simulink model "testmodel"  (R2014b)
settings: Solver=ode3  StartTime=0.0  StopTime=10.0  RelTol=1e-3
settings Model: Creator=Bryan  LastModifiedBy=Bryan
settings RTWCC: TemplateMakefile=RTW.MSVCBuild  Description=Create Visual C/C++ Solution File for Simulink Coder  GenerateReport=on  LaunchReport=on
settings CodeAppCC: ForceParamTrailComments=on  MATLABSourceComments=on
settings GRTTargetCC: MatFileLogging=off

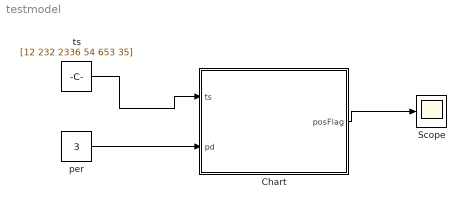
== system testmodel ==
  Chart : Stateflow chart  TreatAsAtomicUnit=on
  Scope : Scope
  "per " : Constant  Value=3
  ts : Constant  Value=[12 232 2336 54 653 35]  VectorParams1D=off
  wires:
  Chart/1(posFlag) -> Scope/1
  ts/1 -> Chart/1(ts)
  "per "/1 -> Chart/2(pd)

== stateflow chart testmodel/Chart ==
  state buy
    en: posFlag=1
  state sell
    en: posFlag=-1
  (default) -> (junction 7) : {avg=testMovAvg(ts,pd)}
  sell -> (junction 7)
  (junction 7) -> sell [order 2] : [avg>50]
  buy -> (junction 7)
  (junction 7) -> buy [order 1] : [avg<50]
  data: x function_input; ped function_input; avgNum function_output; posFlag output size=1; ts input; pd input; avg local
  function avgNum=testMovAvg(x,ped):
    | function avgNum=testMovAvg(x,ped)
    | %ensure out variable does not cofnflict with other model objects 
    | %this directive is need to add input and output on Stateflow chart block!
    | %#codegen
    | avgNum = 0; %must define for code generation
    | avgNum = sum(x)/ped;
